simulink model "Augmentation"  (R2020b)
settings: Solver=VariableStepAuto  StartTime=0.0  StopTime=10.0  RelTol=1e-3
undefined symbols (not defined in the file): B, Beta, ki, kp, M, w0, we, wu
libraries: slpidlib x1
settings Model: Creator=Laura  LastModifiedBy=Laura

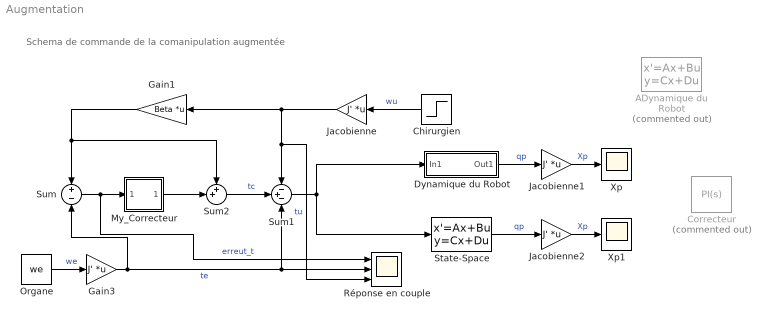
== system Augmentation ==
  note: Schema de commande de la comanipulation augmentée
  ADynamique du Robot : StateSpace  Commented=on  A=M  B=B  C=[1,1]  D=[0,0]  InitialCondition=0
  Chirurgien : Step  Before=w0  After=wu  SampleTime=0  VectorParams1D=off
  Correcteur : slpidlib/PID Controller  Commented=on  Controller=PI  Form=Parallel  TimeDomain=Continuous-time  UseExternalTs=off  SampleTime=-1  IntegratorMethod=Forward Euler  FilterMethod=Forward Euler  ControllerParametersSource=internal  P=kp  I=ki  D=0  UseFilter=on  N=100  TunerSelectOption=Frequency Response Based  InitialConditionSource=internal  InitialConditionForIntegrator=w0  InitialConditionForFilter=0  DifferentiatorICPrevScaledInput=0  ExternalReset=none  TrackingMode=off  Kt=1  LimitOutput=off  SatLimitsSource=internal  UpperSaturationLimit=inf  LowerSaturationLimit=-inf  LinearizeAsGain=on  AntiWindupMode=none  Kb=1  PGainOutDataTypeStr=Inherit: Match scaling  PProdOutDataTypeStr=Inherit: Match scaling  POutMin=[]  POutMax=[]  IGainOutDataTypeStr=Inherit: Match scaling  IProdOutDataTypeStr=Inherit: Match scaling  IOutMin=[]  IOutMax=[]  DOutMin=[]  DOutMax=[]  NOutMin=[]  NOutMax=[]  SumOutDataTypeStr=Inherit: Inherit via back propagation  SumOutMin=[]  SumOutMax=[]  SaturationOutMin=[]  SaturationOutMax=[]  PParamMin=[]  PParamMax=[]  IParamMin=[]  IParamMax=[]  DParamMin=[]  DParamMax=[]  NParamMin=[]  NParamMax=[]  KbParamMin=[]  KbParamMax=[]  KtParamMin=[]  KtParamMax=[]  KbOutMin=[]  KbOutMax=[]  KtOutMin=[]  KtOutMax=[]  IntegratorOutMin=[]  IntegratorOutMax=[]  FilterOutMin=[]  FilterOutMax=[]  SumI1OutMin=[]  SumI1OutMax=[]  SumI2OutMin=[]  SumI2OutMax=[]  SumI3OutMin=[]  SumI3OutMax=[]  SumI4OutMin=[]  SumI4OutMax=[]  SumDOutMin=[]  SumDOutMax=[]  DifferentiatorOutMin=[]  DifferentiatorOutMax=[]  FilterDiffOutCoefMin=[]  FilterDiffOutCoefMax=[]  ReciprocalOutMin=[]  ReciprocalOutMax=[]  SumDenOutMin=[]  SumDenOutMax=[]  SumNumOutMin=[]  SumNumOutMax=[]  DivideOutMin=[]  DivideOutMax=[]  UdiffTsProdOutMin=[]  UdiffTsProdOutMax=[]  NTsProdOutMin=[]  NTsProdOutMax=[]  UintegralTsProdOutMin=[]  UintegralTsProdOutMax=[]  UngainTsProdOutMin=[]  UngainTsProdOutMax=[]  IntegratorContinuousStateAttributes=''  IntegratorStateMustResolveToSignalObject=off  IntegratorRTWStateStorageClass=Auto  FilterContinuousStateAttributes=''  FilterStateMustResolveToSignalObject=off  FilterRTWStateStorageClass=Auto  ParallelPVariant=InternalParameters  IdealPVariant=Disabled  IVariant=InternalParameters  DVariant=Disabled  IntegratorVariant=Continuous  SatVariant=Disabled  AWVariant=Passthrough  PCopyVariant=Disabled  TRVariant=Disabled  FdbkBlocksVariant=Forward  IdealPFdbkVariant=Disabled  SatFdbkVariant=Disabled  DerivativeFilterVariant=Disabled  NVariant=Disabled  NCopyVariant=Disabled_SignalSpec  FilterICVariant=Disabled  IntegratorICVariant=InternalICs  ExternalResetVariant=Disabled  TRSumVariant=Passthrough  SumFdbkVariant=Disabled  SumVariant=Sum_PI  TsampFilterVariant=InternalTs  TsampNgainVariant=Passthrough  TsampIntegralVariant=Passthrough  ExternalSaturationOutDataTypeStr=Inherit: Same as second input
  Dynamique du Robot : Subsystem
      mask Display: disp('(Ms + B)^-1')
  Gain1 : Gain  Gain=Beta  Multiplication=Matrix(K*u)
  Gain3 : Gain  Gain=J'  Multiplication=Matrix(K*u)
  Jacobienne : Gain  Gain=J'  Multiplication=Matrix(K*u)
  Jacobienne1 : Gain  Gain=J'  Multiplication=Matrix(K*u)
  Jacobienne2 : Gain  Gain=J'  Multiplication=Matrix(K*u)
  My_Correcteur : Subsystem
      mask Display: disp('PI')
  Organe : Constant  Value=we  VectorParams1D=off  SampleTime=-1
  Réponse en couple : Scope  NumInputPorts=3
  State-Space : StateSpace  A=-M^-1*B  B=M^-1  C=eye(2)  D=zeros(2,2)  InitialCondition=0
  Sum : Sum  Inputs=+|-
  Sum1 : Sum  Inputs=-+-
  Sum2 : Sum  Inputs=++|
  Xp : Scope
  Xp1 : Scope
  wires:
  Gain3/1 -> Sum/2, Réponse en couple/2, Sum1/3  "te"
  Organe/1 -> Gain3/1  "we"
  Sum1/1 -> Dynamique du Robot/1(In1), State-Space/1
  Dynamique du Robot/1(Out1) -> Jacobienne1/1  "qp"
  Chirurgien/1 -> Jacobienne/1  "wu"
  Jacobienne/1 -> Gain1/1, Réponse en couple/3, Sum1/1  "tu"
  Gain1/1 -> Sum2/1, Sum/1
  Sum2/1 -> Sum1/2  "tc"
  Jacobienne1/1 -> Xp/1  "Xp"
  Sum/1 -> My_Correcteur/1(erreut_t), Réponse en couple/1  "erreut_t"
  My_Correcteur/1(Out1) -> Sum2/2
  Jacobienne2/1 -> Xp1/1  "Xp"
  State-Space/1 -> Jacobienne2/1  "qp"

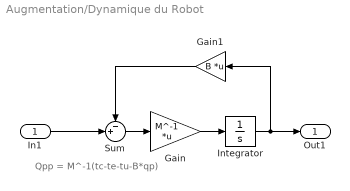
== system Augmentation/Dynamique du Robot ==
  note: Qpp = M^-1(tc-te-tu-B*qp)
  In1 : Inport
  Gain : Gain  Gain=M^-1  Multiplication=Matrix(K*u)
  Gain1 : Gain  Gain=B  Multiplication=Matrix(K*u)
  Integrator : Integrator
  Sum : Sum  Inputs=-+|
  Out1 : Outport
  wires:
  Gain/1 -> Integrator/1
  Sum/1 -> Gain/1
  Gain1/1 -> Sum/1
  Integrator/1 -> Gain1/1, Out1/1
  In1/1 -> Sum/2

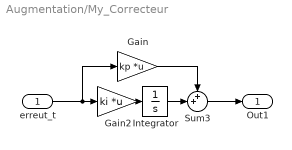
== system Augmentation/My_Correcteur ==
  erreut_t : Inport
  Gain : Gain  Gain=kp  Multiplication=Matrix(K*u)
  Gain2 : Gain  Gain=ki  Multiplication=Matrix(K*u)
  Integrator : Integrator  InitialCondition=w0
  Sum3 : Sum  Inputs=++|
  Out1 : Outport
  wires:
  Sum3/1 -> Out1/1
  Gain/1 -> Sum3/1
  Gain2/1 -> Integrator/1
  Integrator/1 -> Sum3/2
  erreut_t/1 -> Gain/1, Gain2/1
